simulink model "Overcurrent1"  (R2024b)
settings: Solver=VariableStepAuto  StartTime=0.0  StopTime=4  MaxStep=1e-4  RelTol=1e-3
undefined symbols (not defined in the file): D1, Delta
libraries: spsRMSLib x6, simulink_extras x4, spsThreePhaseSeriesRLCBranchLib x2, spsThreePhaseParallelRLCLoadLib x1, spsThreePhaseTransformerTwoWindingsLib x1, spsThreePhaseVIMeasurementLib x1, spsThreePhaseBreakerLib x1, spsThreePhaseFaultLib x1, spsThreePhaseSourceLib x1, sps_lib x1
settings Model: Creator=ADMIN  LastModifiedBy=ADMIN

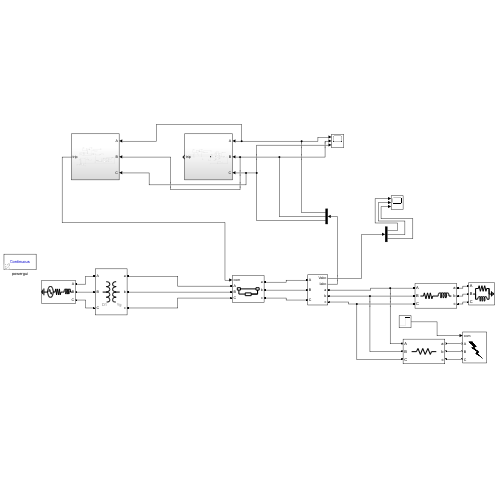
[thumbnail: Simulink's stored preview of the top-level diagram]
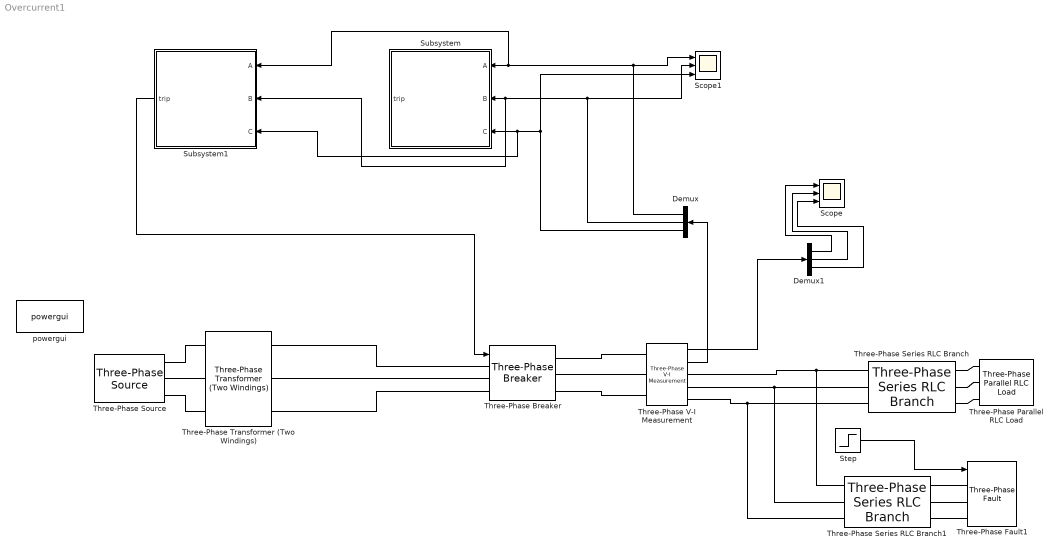
== system Overcurrent1 ==
  Demux : Demux  Outputs=3
  Demux1 : Demux  Outputs=3
  Scope : Scope  NumInputPorts=3
  Scope1 : Scope  NumInputPorts=3
  Step : Step  Time=0.1  After=0.5  SampleTime=0
  Subsystem : Subsystem
  Subsystem1 : Subsystem
  Three-Phase Parallel RLC Load : spsThreePhaseParallelRLCLoadLib/Three-Phase Parallel RLC Load  LConnTagsString=A|B|C  Configuration=Y (grounded)  NominalVoltage=0.4e3  Vabc=[1e3 1e3 1e3]  Vabcp=[1e3 1e3 1e3]  NominalFrequency=50  UnbalancedPower=off  ActivePower=5e6  InductivePower=20e3  CapacitivePower=0  Pabc=[10e3 9e3 11e3]  QLabc=[100 90 110]  QCabc=[100 90 110]  Pabcp=[10e3 9e3 11e3]  QLabcp=[100 90 110]  QCabcp=[100 90 110]  Measurements=None  LoadType=constant Z
  Three-Phase Series RLC Branch : spsThreePhaseSeriesRLCBranchLib/Three-Phase Series RLC Branch  LConnTagsString=A|B|C  RConnTagsString=A|B|C  BranchType=RL  Resistance=0.535  Inductance=0  Capacitance=1e-6  Measurements=None
  Three-Phase Series RLC Branch1 : spsThreePhaseSeriesRLCBranchLib/Three-Phase Series RLC Branch  LConnTagsString=A|B|C  RConnTagsString=A|B|C  BranchType=R  Resistance=0.0485  Inductance=0  Capacitance=1e-6  Measurements=None
  Three-Phase Transformer (Two Windings) : spsThreePhaseTransformerTwoWindingsLib/Three-Phase Transformer (Two Windings)  Winding1Connection=Delta (D1)  Winding2Connection=Yg  CoreType=Three single-phase transformers  SetSaturation=off  Hysteresis=off  DataFile='hysteresis'  SetInitialFlux=off  Measurements=None  UNITS=pu  NominalPower=[ 10e6 , 50 ]  Winding1=[ 11e3 , 0.002 , 0.08 ]  Winding2=[ 0.4e3 , 0.002 , 0.08 ]  Rm=500  Lm=500  L0=0.5  Saturation=[ 0,0 ; 0.0024,1.2 ; 1.0,1.52 ]  InitialFluxes=[ 0.8 , -0.8 , 0.7 ]  BreakLoop=off  DiscreteSolver=Trapezoidal iterative  DataType=off  TransfoNumber=1
  Three-Phase V-I Measurement : spsThreePhaseVIMeasurementLib/Three-Phase V-I Measurement  VoltageMeasurement=phase-to-ground  SetLabelV=off  LabelV=Vabc  Vpu=off  VpuLL=off  CurrentMeasurement=yes  SetLabelI=off  LabelI=Iabc  Ipu=off  Pbase=100e6  Vbase=500e3  OutputType=Complex  PhasorSimulation=off  PSBequivalent=0
  Three-Phase Breaker : spsThreePhaseBreakerLib/Three-Phase Breaker  InitialState=closed  SwitchA=on  SwitchB=on  SwitchC=on  SwitchTimes="[1/60  5/60]"  External=on  BreakerResistance=0.01  SnubberResistance=1e5  SnubberCapacitance=inf  Measurements=None
  Three-Phase Fault1 : spsThreePhaseFaultLib/Three-Phase Fault  InitialStates=0  FaultA=on  FaultB=on  FaultC=on  GroundFault=on  SwitchTimes="[1/60  5/60]"  External=on  SwitchStatus=NaN  FaultResistance=0.001  GroundResistance=0.01  SnubberResistance=1e6  SnubberCapacitance=inf  Measurements=None
  Three-Phase Source : spsThreePhaseSourceLib/Three-Phase Source  InternalConnection=Yg  VoltagePhases=off  Voltage=11e3  PhaseAngle=0  Voltage_phases=[25e3 25e3 25e3]/sqrt(3)  PhaseAngles_phases=[0 -120 +120]  Frequency=50  NonIdealSource=on  SpecifyImpedance=on  Resistance=0.8929  Inductance=16.58e-3  ShortCircuitLevel=20e6  BaseVoltage=11e3  XRratio=7  BusType=swing  Pref=10e6  Qref=0  Prefabc=[10e3, 10e3, 10e3]  Qrefabc=[0, 0, 0]  Qmin=-inf  Qmax=inf
  powergui : sps_lib/powergui  Priority=1  SimulationMode=Continuous  SampleTime=50e-6  frequency=60  Iterations=50  frequencyindice=50  Pbase=100e6  ErrMax=1e-4  UnitsV=kV  UnitsW=MW  buscounter=0  FunctionMessages=off  echomessages=off  EnableUseOfTLC=off  CurrentSourceSwitches=off  DisableSnubberDevices=off  DisableRonSwitches=off  DisableVfSwitches=off  DisplayEquations=off  AutomaticDiscreteSolvers=off  SolverType=Tustin/Backward Euler (TBE)  Interpol=off  ExternalGateDelay=off  methode=off  Ts=100  x0status=blocks  SPID=on  SwTol=0  HookPort=off  NonlinearTolerance=1e-4  nMaxIteration=100  ContinueOnMaxIteration=off  RestoreLinks=warning  ResistiveCurrentMeasurement=off  Frange=[0:2:500]  Ylog=off  Xlog=on  ShowGrid=off  save=off  variable=ZData  structure=0  ZoomFFT=off  StartTime=0.0  cycles=1  DisplayStyle=1  fundamental=60  FreqAxis=off  MaxFrequency=1000  frequencyindicesteady=1  RmsSteady=1  display=off
  wires:
  Demux1/3 -> Scope/3
  Three-Phase V-I Measurement/2 -> Demux/1
  Demux/1 -> Scope1/1, Subsystem1/1(A), Subsystem/1(A)
  Demux/3 -> Scope1/3, Subsystem1/3(C), Subsystem/3(C)
  Demux/2 -> Scope1/2, Subsystem1/2(B), Subsystem/2(B)
  Demux1/2 -> Scope/2
  Three-Phase V-I Measurement/1 -> Demux1/1
  Demux1/1 -> Scope/1
  Step/1 -> Three-Phase Fault1/1
  Subsystem1/1(trip) -> Three-Phase Breaker/1
  connections:
  Three-Phase Series RLC Branch/LConn3 -- Three-Phase Series RLC Branch1/LConn3 -- Three-Phase V-I Measurement/RConn3
  Three-Phase V-I Measurement/RConn2 -- Three-Phase Series RLC Branch1/LConn2 -- Three-Phase Series RLC Branch/LConn2
  Three-Phase V-I Measurement/RConn1 -- Three-Phase Series RLC Branch1/LConn1 -- Three-Phase Series RLC Branch/LConn1
  Three-Phase V-I Measurement/LConn1 -- Three-Phase Breaker/RConn1
  Three-Phase Transformer (Two Windings)/RConn1 -- Three-Phase Breaker/LConn1
  Three-Phase Breaker/LConn2 -- Three-Phase Transformer (Two Windings)/RConn2
  Three-Phase Source/RConn3 -- Three-Phase Transformer (Two Windings)/LConn3
  Three-Phase Transformer (Two Windings)/RConn3 -- Three-Phase Breaker/LConn3
  Three-Phase Source/RConn2 -- Three-Phase Transformer (Two Windings)/LConn2
  Three-Phase Source/RConn1 -- Three-Phase Transformer (Two Windings)/LConn1
  Three-Phase V-I Measurement/LConn2 -- Three-Phase Breaker/RConn2
  Three-Phase Breaker/RConn3 -- Three-Phase V-I Measurement/LConn3
  Three-Phase Series RLC Branch/RConn1 -- Three-Phase Parallel RLC Load/LConn1
  Three-Phase Series RLC Branch/RConn2 -- Three-Phase Parallel RLC Load/LConn2
  Three-Phase Series RLC Branch/RConn3 -- Three-Phase Parallel RLC Load/LConn3
  Three-Phase Fault1/LConn1 -- Three-Phase Series RLC Branch1/RConn1
  Three-Phase Fault1/LConn2 -- Three-Phase Series RLC Branch1/RConn2
  Three-Phase Fault1/LConn3 -- Three-Phase Series RLC Branch1/RConn3

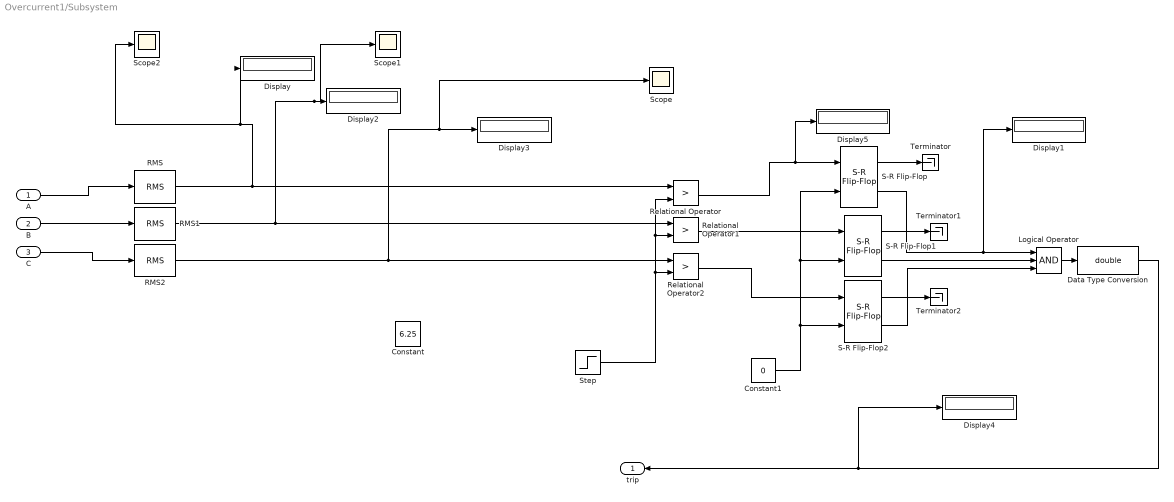
== system Overcurrent1/Subsystem ==
  A : Inport
  B : Inport  Port=2
  C : Inport  Port=3
  Constant : Constant  Value=6.25
  Constant1 : Constant  Value=0  OutDataTypeStr=boolean
  Data Type Conversion : DataTypeConversion  OutDataTypeStr=double  SaturateOnIntegerOverflow=off  RndMeth=Floor
  Display{,1..5} (6 alike) : Display
  Logical Operator : Logic  Inputs=3  AllPortsSameDT=off  OutDataTypeStr=boolean
  RMS : spsRMSLib/RMS  TrueRMS=on  Freq=50  RMSInit=0  Ts=0
  RMS1 : spsRMSLib/RMS  TrueRMS=on  Freq=50  RMSInit=0  Ts=0
  RMS2 : spsRMSLib/RMS  TrueRMS=on  Freq=50  RMSInit=0  Ts=0
  Relational Operator : RelationalOperator  Operator=>  OutDataTypeStr=boolean  RndMeth=Simplest  InputSameDT=off
  Relational Operator1 : RelationalOperator  Operator=>  OutDataTypeStr=boolean  RndMeth=Simplest  InputSameDT=off
  Relational Operator2 : RelationalOperator  Operator=>  OutDataTypeStr=boolean  RndMeth=Simplest  InputSameDT=off
  S-R Flip-Flop : simulink_extras/Flip Flops/S-R Flip-Flop  initial_condition=0
  S-R Flip-Flop1 : simulink_extras/Flip Flops/S-R Flip-Flop  initial_condition=0
  S-R Flip-Flop2 : simulink_extras/Flip Flops/S-R Flip-Flop  initial_condition=0
  Scope : Scope
  Scope1 : Scope
  Scope2 : Scope
  Step : Step  Time=1.4  Before=11e3  SampleTime=0
  Terminator : Terminator
  Terminator1 : Terminator
  Terminator2 : Terminator
  trip : Outport
  wires:
  S-R Flip-Flop1/1 -> Terminator1/1
  Logical Operator/1 -> Data Type Conversion/1
  S-R Flip-Flop/1 -> Terminator/1
  S-R Flip-Flop2/2 -> Logical Operator/3
  Relational Operator2/1 -> S-R Flip-Flop2/1
  C/1 -> RMS2/1
  Constant1/1 -> S-R Flip-Flop2/2, S-R Flip-Flop/2, S-R Flip-Flop1/2
  Relational Operator1/1 -> S-R Flip-Flop1/1
  Step/1 -> Relational Operator1/2, Relational Operator/2, Relational Operator2/2
  S-R Flip-Flop/2 -> Display1/1, Logical Operator/1
  Data Type Conversion/1 -> Display4/1, trip/1
  B/1 -> RMS1/1
  Relational Operator/1 -> Display5/1, S-R Flip-Flop/1
  S-R Flip-Flop2/1 -> Terminator2/1
  S-R Flip-Flop1/2 -> Logical Operator/2
  A/1 -> RMS/1
  RMS/1 -> Scope2/1, Display/1, Relational Operator/1
  RMS1/1 -> Scope1/1, Display2/1, Relational Operator1/1
  RMS2/1 -> Scope/1, Display3/1, Relational Operator2/1

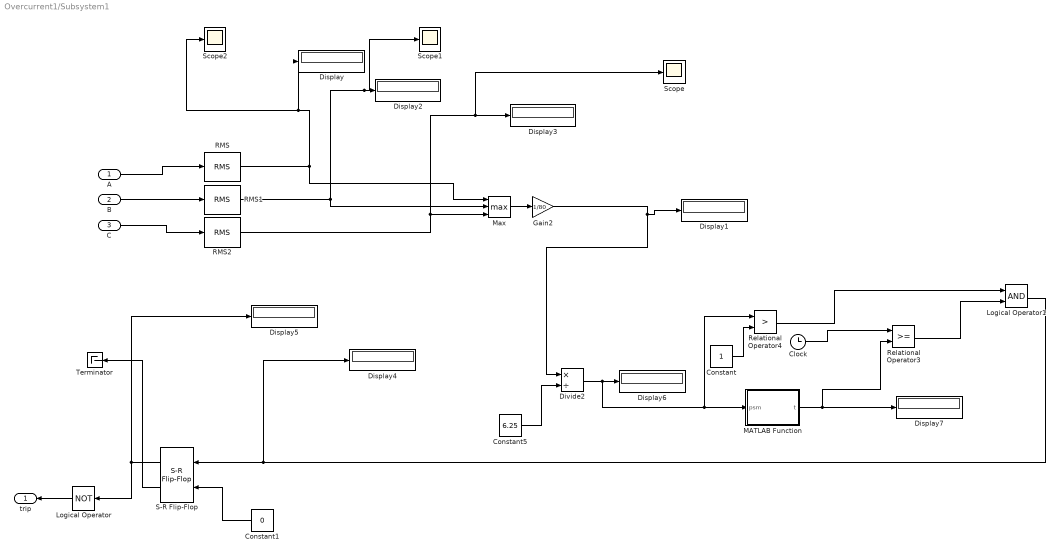
== system Overcurrent1/Subsystem1 ==
  A : Inport
  B : Inport  Port=2
  C : Inport  Port=3
  Clock : Clock
  Constant : Constant
  Constant1 : Constant  Value=0  OutDataTypeStr=boolean
  Constant5 : Constant  Value=6.25
  Display{,1..7} (8 alike) : Display
  Divide2 : Product  Inputs=*/
  Gain2 : Gain  Gain=1/80
  Logical Operator : Logic  Operator=NOT  AllPortsSameDT=off  OutDataTypeStr=boolean
  Logical Operator1 : Logic  AllPortsSameDT=off  OutDataTypeStr=boolean
  MATLAB Function : MATLAB Function  TreatAsAtomicUnit=on
  Max : MinMax  Function=max  Inputs=3
  RMS : spsRMSLib/RMS  TrueRMS=on  Freq=50  RMSInit=0  Ts=0
  RMS1 : spsRMSLib/RMS  TrueRMS=on  Freq=50  RMSInit=0  Ts=0
  RMS2 : spsRMSLib/RMS  TrueRMS=on  Freq=50  RMSInit=0  Ts=0
  Relational Operator3 : RelationalOperator  OutDataTypeStr=boolean  RndMeth=Simplest  InputSameDT=off
  Relational Operator4 : RelationalOperator  Operator=>  OutDataTypeStr=boolean  RndMeth=Simplest  InputSameDT=off
  S-R Flip-Flop : simulink_extras/Flip Flops/S-R Flip-Flop  initial_condition=0
  Scope : Scope
  Scope1 : Scope
  Scope2 : Scope
  Terminator : Terminator
  trip : Outport
  wires:
  C/1 -> RMS2/1
  B/1 -> RMS1/1
  A/1 -> RMS/1
  RMS2/1 -> Scope/1, Display3/1, Max/3
  RMS/1 -> Scope2/1, Display/1, Max/1
  Constant5/1 -> Divide2/2
  RMS1/1 -> Scope1/1, Display2/1, Max/2
  Divide2/1 -> Relational Operator4/1, MATLAB Function/1(psm), Display6/1
  Clock/1 -> Relational Operator3/1
  Constant/1 -> Relational Operator4/2
  Relational Operator4/1 -> Logical Operator1/1
  Max/1 -> Gain2/1
  Gain2/1 -> Divide2/1, Display1/1
  MATLAB Function/1(t) -> Relational Operator3/2, Display7/1
  Relational Operator3/1 -> Logical Operator1/2
  Logical Operator1/1 -> Display4/1, S-R Flip-Flop/1
  Constant1/1 -> S-R Flip-Flop/2
  S-R Flip-Flop/1 -> Display5/1, Logical Operator/1
  S-R Flip-Flop/2 -> Terminator/1
  Logical Operator/1 -> trip/1

== matlab function Overcurrent1/Subsystem1/MATLAB Function ==
  data: psm input; t output
function t=idmt(psm)
TMS=0.5;
if psm<=1
    t=inf;
else
    t=0.1+3.2*TMS;
end
